simulink model "d_sim"  (R2024a)
settings: Solver=ode4  StartTime=0.0  StopTime=10.0  FixedStep=0.01  RelTol=1e-3
libraries: matrix_library x2, simulink_extras x1, aerolibutil x1
settings Model: SnapshotInterval=1  Creator=vd662f  LastModifiedBy=gladstonjoseph
settings SolverCC: AlgebraicLoopSolver=TrustRegion
settings DataIOCC: ReturnWorkspaceOutputs=off
settings DebuggingCC: UnconnectedInputMsg=warning  UnconnectedOutputMsg=warning  UnconnectedLineMsg=warning  ArithmeticOperatorsInVariantConditions=warning
settings ModelReferenceCC: EnableRefExpFcnMdlSchedulingChecks=on
settings SFSimCC: SimUseLocalCustomCode=off  CustomCodeUndefinedFunction=UseInterfaceOnly
settings RTWCC: RTWUseLocalCustomCode=off  GPUComputeCapability=3.5

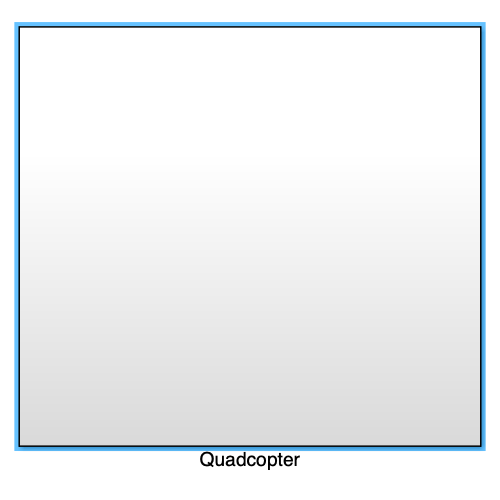
[thumbnail: Simulink's stored preview of the top-level diagram]
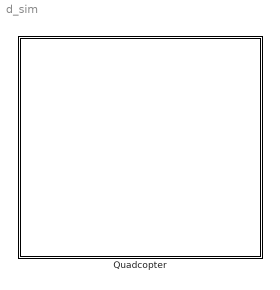
== system d_sim ==
  Quadcopter : Subsystem

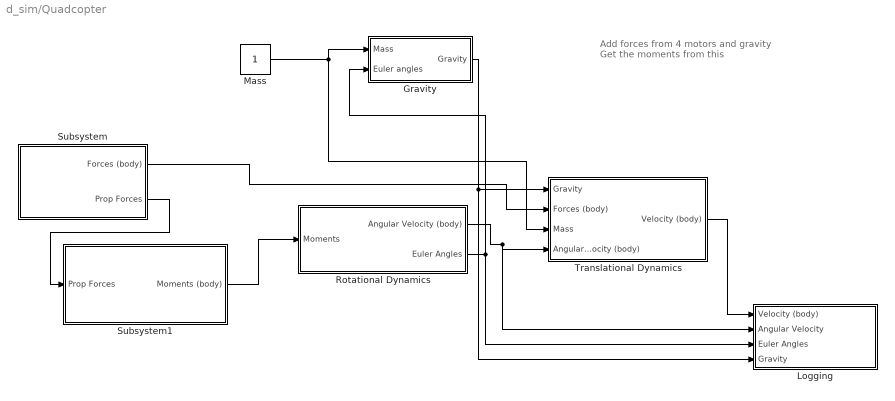
== system d_sim/Quadcopter ==
  note: Add forces from 4 motors and gravity
      | Get the moments from this
  Gravity : Subsystem
  Logging : Subsystem
  Mass : Constant
  Rotational Dynamics : Subsystem
  Subsystem : Subsystem
  Subsystem1 : Subsystem
  Translational Dynamics : Subsystem
  wires:
  Mass/1 -> Gravity/1(Mass), Translational Dynamics/3(Mass)
  Subsystem/1(Forces (body)) -> Translational Dynamics/2(Forces (body))
  Subsystem1/1(Moments (body)) -> Rotational Dynamics/1(Moments)
  Rotational Dynamics/1(Angular Velocity (body)) -> Logging/2(Angular Velocity), Translational Dynamics/4(Angular Velocity (body))
  Gravity/1(Gravity) -> Translational Dynamics/1(Gravity), Logging/4(Gravity)
  Rotational Dynamics/2(Euler Angles) -> Gravity/2(Euler angles), Logging/3(Euler Angles)
  Translational Dynamics/1(Velocity (body)) -> Logging/1(Velocity (body))
  Subsystem/2(Prop Forces) -> Subsystem1/1(Prop Forces)

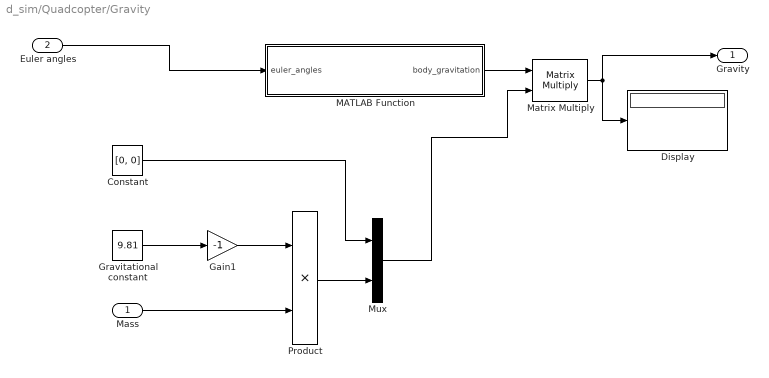
== system d_sim/Quadcopter/Gravity ==
  Mass : Inport
  Euler angles : Inport  Port=2
  Constant : Constant  Value=[0, 0]
  Display : Display
  Gain1 : Gain  Gain=-1
  Gravitational constant : Constant  Value=9.81
  MATLAB Function : MATLAB Function  TreatAsAtomicUnit=on
  Matrix Multiply : Product  Multiplication=Matrix(*)
  Mux : Mux  Inputs=2
  Product : Product
  Gravity : Outport  VectorParamsAs1DForOutWhenUnconnected=off
  wires:
  Mass/1 -> Product/2
  Gain1/1 -> Product/1
  Gravitational constant/1 -> Gain1/1
  Product/1 -> Mux/2
  Constant/1 -> Mux/1
  Mux/1 -> Matrix Multiply/2
  MATLAB Function/1(body_gravitation) -> Matrix Multiply/1
  Euler angles/1 -> MATLAB Function/1(euler_angles)
  Matrix Multiply/1 -> Display/1, Gravity/1

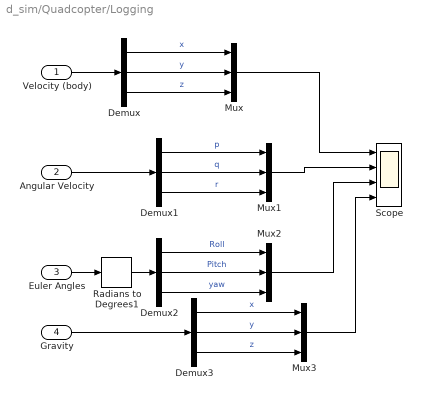
== system d_sim/Quadcopter/Logging ==
  Velocity (body) : Inport
  Angular Velocity : Inport  Port=2
  Euler Angles : Inport  Port=3
  Gravity : Inport  Port=4
  Demux{,1..3} (4 alike) : Demux  Outputs=3
  Mux{,1..3} (4 alike) : Mux  Inputs=3
  Radians to Degrees1 : simulink_extras/Transformations/Radians to Degrees
  Scope : Scope  NumInputPorts=4
  wires:
  Velocity (body)/1 -> Demux/1
  Demux/1 -> Mux/1  "x"
  Demux/2 -> Mux/2  "y"
  Demux/3 -> Mux/3  "z"
  Demux1/3 -> Mux1/3  "r"
  Demux1/2 -> Mux1/2  "q"
  Demux1/1 -> Mux1/1  "p"
  Angular Velocity/1 -> Demux1/1
  Euler Angles/1 -> Radians to Degrees1/1
  Demux2/1 -> Mux2/1  "Roll"
  Demux2/2 -> Mux2/2  "Pitch"
  Demux2/3 -> Mux2/3  "yaw"
  Mux/1 -> Scope/1
  Mux1/1 -> Scope/2
  Mux2/1 -> Scope/3
  Radians to Degrees1/1 -> Demux2/1
  Mux3/1 -> Scope/4
  Gravity/1 -> Demux3/1
  Demux3/1 -> Mux3/1  "x"
  Demux3/2 -> Mux3/2  "y"
  Demux3/3 -> Mux3/3  "z"

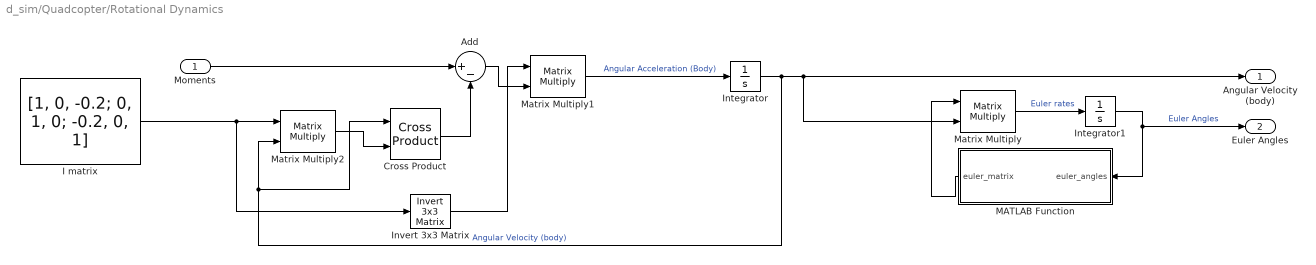
== system d_sim/Quadcopter/Rotational Dynamics ==
  Moments : Inport
  Add : Sum  Inputs=|+-
  Cross Product : matrix_library/Cross Product
  I matrix : Constant  Value=[1, 0, -0.2; 0, 1, 0; -0.2, 0, 1]
  Integrator : Integrator  InitialCondition=[0; 0; 0]
  Integrator1 : Integrator  InitialCondition=[0; 0; 0]
  Invert 3x3 Matrix : aerolibutil/Invert  3x3 Matrix
  MATLAB Function : MATLAB Function  TreatAsAtomicUnit=on
  Matrix Multiply : Product  Multiplication=Matrix(*)
  Matrix Multiply1 : Product  Multiplication=Matrix(*)
  Matrix Multiply2 : Product  Multiplication=Matrix(*)
  Angular Velocity (body) : Outport
  Euler Angles : Outport  Port=2
  wires:
  Matrix Multiply1/1 -> Integrator/1  "Angular Acceleration (Body)"
  Invert 3x3 Matrix/1 -> Matrix Multiply1/1
  Integrator/1 -> Angular Velocity (body)/1, Matrix Multiply/2, Cross Product/1, Matrix Multiply2/2  "Angular Velocity (body)"
  I matrix/1 -> Matrix Multiply2/1, Invert 3x3 Matrix/1
  Matrix Multiply/1 -> Integrator1/1  "Euler rates"
  Integrator1/1 -> MATLAB Function/1(euler_angles), Euler Angles/1  "Euler Angles"
  MATLAB Function/1(euler_matrix) -> Matrix Multiply/1
  Moments/1 -> Add/1
  Matrix Multiply2/1 -> Cross Product/2
  Add/1 -> Matrix Multiply1/2
  Cross Product/1 -> Add/2

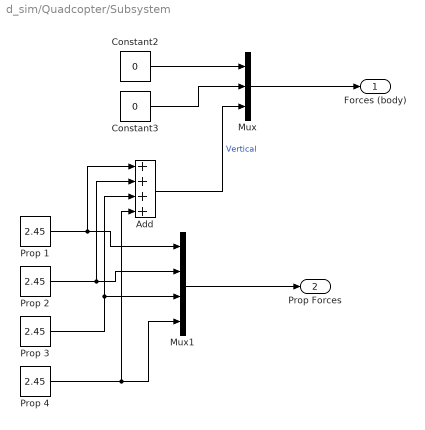
== system d_sim/Quadcopter/Subsystem ==
  Add : Sum  Inputs=++++
  Constant2 : Constant  Value=0
  Constant3 : Constant  Value=0
  Mux : Mux  Inputs=3
  Mux1 : Mux
  Prop {1..4} (4 alike) : Constant  Value=2.45
  Forces (body) : Outport
  Prop Forces : Outport  Port=2
  wires:
  Constant2/1 -> Mux/1
  Mux/1 -> Forces (body)/1
  Constant3/1 -> Mux/2
  Add/1 -> Mux/3  "Vertical"
  Mux1/1 -> Prop Forces/1
  Prop 1/1 -> Add/1, Mux1/1
  Prop 2/1 -> Add/2, Mux1/2
  Prop 3/1 -> Mux1/3, Add/3
  Prop 4/1 -> Add/4, Mux1/4

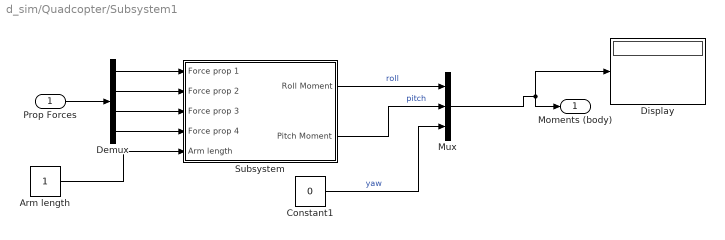
== system d_sim/Quadcopter/Subsystem1 ==
  Prop Forces : Inport
  Arm length : Constant
  Constant1 : Constant  Value=0
  Demux : Demux
  Display : Display
  Mux : Mux  Inputs=3
  Subsystem : Subsystem
  Moments (body) : Outport
  wires:
  Constant1/1 -> Mux/3  "yaw"
  Subsystem/2(Pitch Moment) -> Mux/2  "pitch"
  Mux/1 -> Display/1, Moments (body)/1
  Subsystem/1(Roll Moment) -> Mux/1  "roll"
  Prop Forces/1 -> Demux/1
  Demux/1 -> Subsystem/1(Force prop 1)
  Demux/2 -> Subsystem/2(Force prop 2)
  Demux/3 -> Subsystem/3(Force prop 3)
  Demux/4 -> Subsystem/4(Force prop 4)
  Arm length/1 -> Subsystem/5(Arm length)

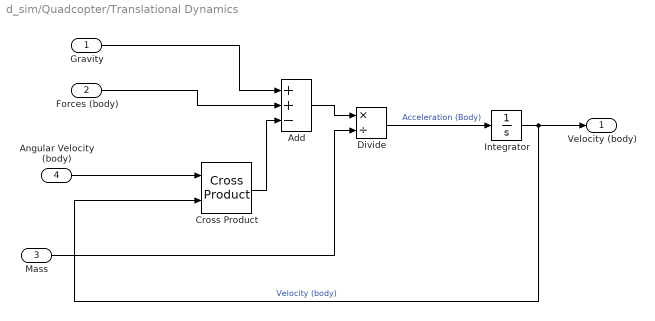
== system d_sim/Quadcopter/Translational Dynamics ==
  Gravity : Inport
  Forces (body) : Inport  Port=2
  Mass : Inport  Port=3
  Angular Velocity (body) : Inport  Port=4
  Add : Sum  Inputs=++-
  Cross Product : matrix_library/Cross Product
  Divide : Product  Inputs=*/
  Integrator : Integrator  InitialCondition=[0; 0; 0]
  Velocity (body) : Outport
  wires:
  Forces (body)/1 -> Add/2
  Cross Product/1 -> Add/3
  Integrator/1 -> Cross Product/2, Velocity (body)/1  "Velocity (body)"
  Add/1 -> Divide/1
  Mass/1 -> Divide/2
  Divide/1 -> Integrator/1  "Acceleration (Body)"
  Angular Velocity (body)/1 -> Cross Product/1
  Gravity/1 -> Add/1

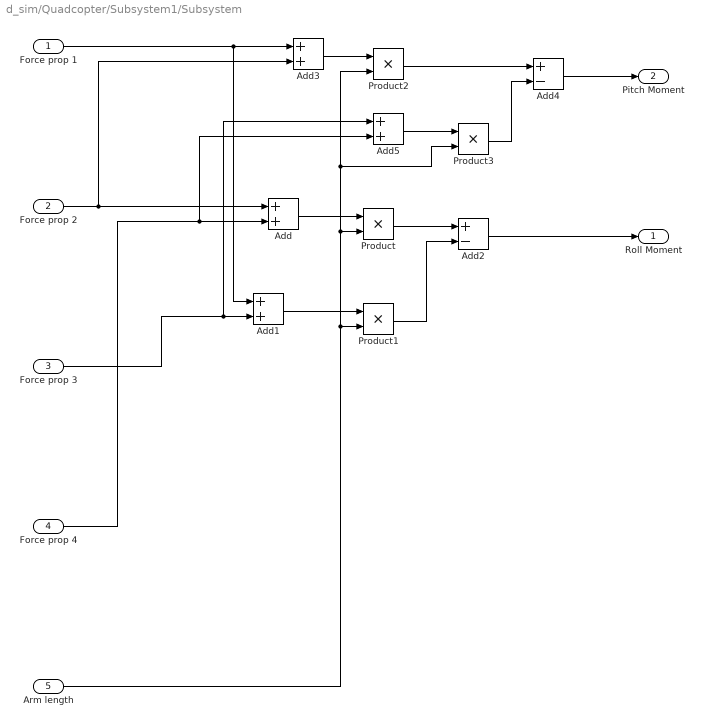
== system d_sim/Quadcopter/Subsystem1/Subsystem ==
  Force prop 1 : Inport
  Force prop 2 : Inport  Port=2
  Force prop 3 : Inport  Port=3
  Force prop 4 : Inport  Port=4
  Arm length : Inport  Port=5
  Add{,1,3,5} (4 alike) : Sum
  Add2 : Sum  Inputs=+-
  Add4 : Sum  Inputs=+-
  Product{,1..3} (4 alike) : Product
  Roll Moment : Outport
  Pitch Moment : Outport  Port=2
  wires:
  Force prop 2/1 -> Add3/2, Add/1
  Force prop 4/1 -> Add5/2, Add/2
  Add/1 -> Product/1
  Arm length/1 -> Product3/2, Product2/2, Product/2, Product1/2
  Force prop 1/1 -> Add3/1, Add1/1
  Force prop 3/1 -> Add5/1, Add1/2
  Add1/1 -> Product1/1
  Product/1 -> Add2/1
  Product1/1 -> Add2/2
  Add2/1 -> Roll Moment/1
  Add3/1 -> Product2/1
  Product2/1 -> Add4/1
  Add5/1 -> Product3/1
  Product3/1 -> Add4/2
  Add4/1 -> Pitch Moment/1

== matlab function d_sim/Quadcopter/Rotational Dynamics/MATLAB Function ==
  data: euler_angles input; euler_matrix output
function euler_matrix = get_matrix(euler_angles)

    phi = euler_angles(1);
    theta = euler_angles(2);
    psi = euler_angles(3);

    euler_matrix = [1, sin(phi)*tan(theta), cos(phi)*tan(theta);...
                    0, cos(phi), -sin(phi);...
                    0, sin(phi)*sec(theta), cos(phi)*sec(theta)];

end

== matlab function d_sim/Quadcopter/Gravity/MATLAB Function ==
  data: euler_angles input; body_gravitation output
function body_gravitation = gravity_matrix(euler_angles)

    phi = euler_angles(1);
    theta = euler_angles(2);
    psi = euler_angles(3);

    body_gravitation = [cos(theta)*cos(psi), cos(theta)*sin(psi), -sin(theta);...
                        sin(phi)*sin(theta)*cos(psi) - cos(phi)*sin(psi), sin(phi)*sin(theta)*sin(psi) + cos(phi)*cos(psi), sin(phi)*cos(theta);...
                        cos(phi)*sin(theta)*cos(psi) + sin(phi)*sin(psi), cos(phi)*sin(theta)*sin(psi) + sin(phi)*cos(psi), cos(phi)*cos(theta)];

end
